simulink model "untitled1"  (R2021a)
settings: Solver=VariableStepAuto  StartTime=0.0  StopTime=t_end  FixedStep=sim_step  RelTol=1e-3
values from neighbouring files (symbols this model uses):
  a1 = Teta22(1,end)    [projekat_skripta.m]
  N_reg = 10    [projekat_skripta.m]
  t_bp = 250    [projekat_skripta.m]
  t_prbs = 250    [projekat_skripta.m]
  T_prekidanje = 10    [projekat_skripta.m]
  T_samp = t_resampled(2) - t_resampled(1)    [projekat_skripta.m]
  t_step_vent = 200    [projekat_skripta.m]
  u_max = 3    [projekat_skripta.m]
  u_nom_temp = 4.5    [projekat_skripta.m]
  u_nom_vent = 6    [projekat_skripta.m]
  u_step_vent = 3    [projekat_skripta.m]
undefined symbols (not defined in the file or in its folder): National_Instruments, PCIe
libraries: sldrtlib x4
settings Model: Creator=lab  LastModifiedBy=bd200090d

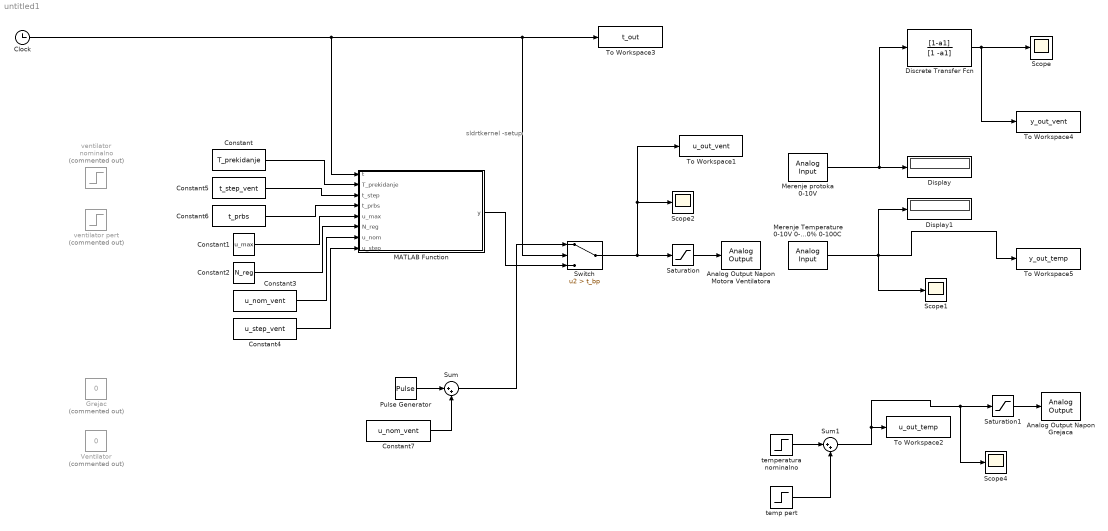
== system untitled1 ==
  note: sldrtkernel -setup
  Analog Output Napon Grejaca : sldrtlib/Analog Output  SampleTime=0.01  MaxMissedTicks=10000  ShowMissedTicks=off  YieldWhenWaiting=off  DrvName=National_Instruments/PCIe-6323  DrvAddress=4294967295  DrvOptions=[0 0 0 0 0 0 0]  Channels=2  RangeMode=1  VoltRange=1  InitialValue=0  FinalValue=0
      settings: AttributesFormatString=National Instruments\nPCIe-6323 [auto]
  Analog Output Napon Motora Ventilatora : sldrtlib/Analog Output  SampleTime=0.01  MaxMissedTicks=10000  ShowMissedTicks=off  YieldWhenWaiting=off  DrvName=National_Instruments/PCIe-6323  DrvAddress=4294967295  DrvOptions=[0 0 0 0 0 0 0]  Channels=1  RangeMode=1  VoltRange=1  InitialValue=[]  FinalValue=[]
      settings: AttributesFormatString=National Instruments\nPCIe-6323 [auto]
  Clock : Clock
  Constant : Constant  Value=T_prekidanje
  Constant1 : Constant  Value=u_max
  Constant2 : Constant  Value=N_reg
  Constant3 : Constant  Value=u_nom_vent
  Constant4 : Constant  Value=u_step_vent
  Constant5 : Constant  Value=t_step_vent
  Constant6 : Constant  Value=t_prbs
  Constant7 : Constant  Value=u_nom_vent
  Discrete Transfer Fcn : DiscreteTransferFcn  Numerator=[1-a1]  Denominator=[1 -a1]
  Display : Display
  Display1 : Display
  Grejac : Constant  Commented=on  Value=0
  MATLAB Function : MATLAB Function  TreatAsAtomicUnit=on
  Merenje Temperature 0-10V 0-100% 0-100C : sldrtlib/Analog Input  SampleTime=0.01  MaxMissedTicks=10000  ShowMissedTicks=off  YieldWhenWaiting=off  DrvName=National_Instruments/PCIe-6323  DrvAddress=4294967295  DrvOptions=[0 0 0 0 0 0 0]  Channels=3  RangeMode=1  VoltRange=1  DataType=1
      settings: AttributesFormatString=National Instruments\nPCIe-6323 [auto]
  Merenje protoka 0-10V : sldrtlib/Analog Input  SampleTime=0.01  MaxMissedTicks=10000  ShowMissedTicks=off  YieldWhenWaiting=on  DrvName=National_Instruments/PCIe-6323  DrvAddress=4294967295  DrvOptions=[0 0 0 0 0 0 0]  Channels=6  RangeMode=1  VoltRange=1  DataType=1
      settings: AttributesFormatString=National Instruments\nPCIe-6323 [auto]
  Pulse Generator : DiscretePulseGenerator  PulseType=Time based  Amplitude=u_max  Period=2*T_prekidanje  PulseWidth=50
  Saturation : Saturate  UpperLimit=10  LowerLimit=0
  Saturation1 : Saturate  UpperLimit=10  LowerLimit=0
  Scope{,1..2,4} (4 alike) : Scope
  Sum : Sum  Inputs=|++
  Sum1 : Sum  Inputs=|++
  Switch : Switch  Criteria=u2 > Threshold  Threshold=t_bp
  To Workspace1 : ToWorkspace  VariableName=u_out_vent  SaveFormat=Timeseries  SampleTime=T_samp
  To Workspace2 : ToWorkspace  VariableName=u_out_temp  SaveFormat=Timeseries  SampleTime=-1
  To Workspace3 : ToWorkspace  VariableName=t_out  SaveFormat=Timeseries  SampleTime=-1
  To Workspace4 : ToWorkspace  VariableName=y_out_vent  SaveFormat=Timeseries  SampleTime=T_samp
  To Workspace5 : ToWorkspace  VariableName=y_out_temp  SaveFormat=Timeseries  SampleTime=-1
  Ventilator : Constant  Commented=on  Value=0
  temp pert : Step  Time=0  After=0  SampleTime=0  ZeroCross=off
  temperatura nominalno : Step  Time=0  After=u_nom_temp  SampleTime=0
  ventilator nominalno : Step  Commented=on  Time=5  After=u_nom_vent  SampleTime=0
  ventilator pert : Step  Commented=on  Time=t_step_vent  After=u_step_vent  SampleTime=0
  wires:
  Sum1/1 -> Scope4/1, Saturation1/1, To Workspace2/1
  Saturation1/1 -> Analog Output Napon Grejaca/1
  Merenje protoka 0-10V/1 -> Discrete Transfer Fcn/1, Display/1
  Saturation/1 -> Analog Output Napon Motora Ventilatora/1
  MATLAB Function/1(y) -> Switch/3
  Merenje Temperature 0-10V 0-100% 0-100C/1 -> Scope1/1, Display1/1, To Workspace5/1
  temperatura nominalno/1 -> Sum1/1
  temp pert/1 -> Sum1/2
  Constant/1 -> MATLAB Function/2(T_prekidanje)
  Constant1/1 -> MATLAB Function/5(u_max)
  Constant2/1 -> MATLAB Function/6(N_reg)
  Constant3/1 -> MATLAB Function/7(u_nom)
  Discrete Transfer Fcn/1 -> To Workspace4/1, Scope/1
  Constant4/1 -> MATLAB Function/8(u_step)
  Constant5/1 -> MATLAB Function/3(t_step)
  Constant6/1 -> MATLAB Function/4(t_prbs)
  Clock/1 -> Switch/2, To Workspace3/1, MATLAB Function/1(t)
  Pulse Generator/1 -> Sum/1
  Constant7/1 -> Sum/2
  Sum/1 -> Switch/1
  Switch/1 -> To Workspace1/1, Scope2/1, Saturation/1

== matlab function untitled1/MATLAB Function ==
  data: t input; y output; T_prekidanje input; t_step input; t_prbs input; u_max input; N_reg input; u_nom input; u_step input
function y = PRBS(t, T_prekidanje, t_step, t_prbs, u_max, N_reg, u_nom, u_step)
    persistent reg
    
    if (isempty(reg))
       reg = ones(1,N_reg); 
    end
    
    if (t <= t_step)
        y = u_nom;
    elseif ((t > t_step) && (t < t_prbs))
        y = u_nom + u_step;
    else 
        if (mod(t,T_prekidanje)==0)
            temp = mod(reg(2)+reg(6)+reg(3)+reg(9),2);

            reg = [temp reg(1:N_reg-1)];

        end
        y = u_max*reg(1) + u_nom ; 
    end
end
